simulink model "physical_dynamics_transfer_model"  (R2012b)
settings: Solver=ode1  StartTime=0.0  StopTime=10  FixedStep=0.002  RelTol=1e-3
undefined symbols (not defined in the file or in its folder): HIL, x_init
libraries: quarc_library x4
settings Model: ExtModeTrigDuration=5000  Creator=crbonney  LastModifiedBy=crbonney
settings SolverCC: PositivePriorityOrder=on
settings RTWCC: SystemTargetFile=quarc_win64.tlc  TemplateMakefile=quarc_default_tmf  Description=QUARC Win64 Target  ProcessScript=quarc_win64_make_rtw_hook
settings STFCustomTargetCC: TargetPreCompLibLocation=C:\PROGRA~3\QUARC\lib\2012b\win64\release  CodeReplacementLibrary=ANSI_C  GeneratePreprocessorConditionals=Disable all  CombineOutputUpdateFcns=on  GRTInterface=off  SystemTargetFile=quarc_win64.tlc
settings GRTTargetCC: TargetPreCompLibLocation=C:\PROGRA~3\QUARC\lib\2012b\win64\release  ParMdlRefBuildCompliant=off  CompOptLevelCompliant=off  ConcurrentExecutionCompliant=off  MatFileLogging=off  ExtMode=on  ExtModeMexFile=quarc_comm

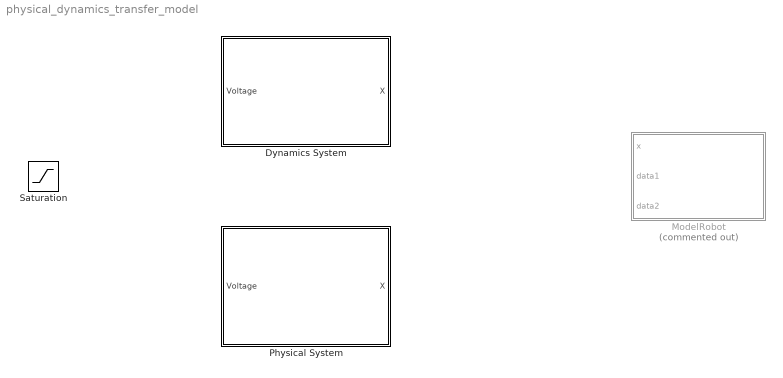
== system physical_dynamics_transfer_model ==
  Dynamics System : Subsystem
  ModelRobot : MATLAB Function  Commented=on  TreatAsAtomicUnit=on
  Physical System : Subsystem
  Saturation : Saturate  UpperLimit=10  LowerLimit=-10
  wires:
  ? -> Saturation/1  "Input V"

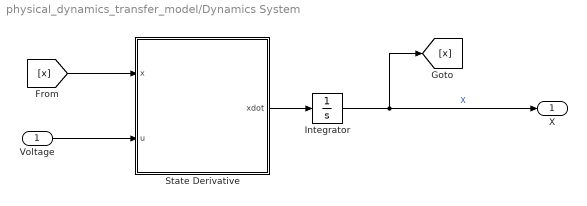
== system physical_dynamics_transfer_model/Dynamics System ==
  Voltage : Inport
  Integrator : Integrator  InitialCondition=x_init
  State Derivative : MATLAB Function  TreatAsAtomicUnit=on
  X : Outport
  wires:
  State Derivative/1(xdot) -> Integrator/1
  Voltage/1 -> State Derivative/2(u)
  [x] -> State Derivative/1(x)
  Integrator/1 -> X/1, [x]  "X"

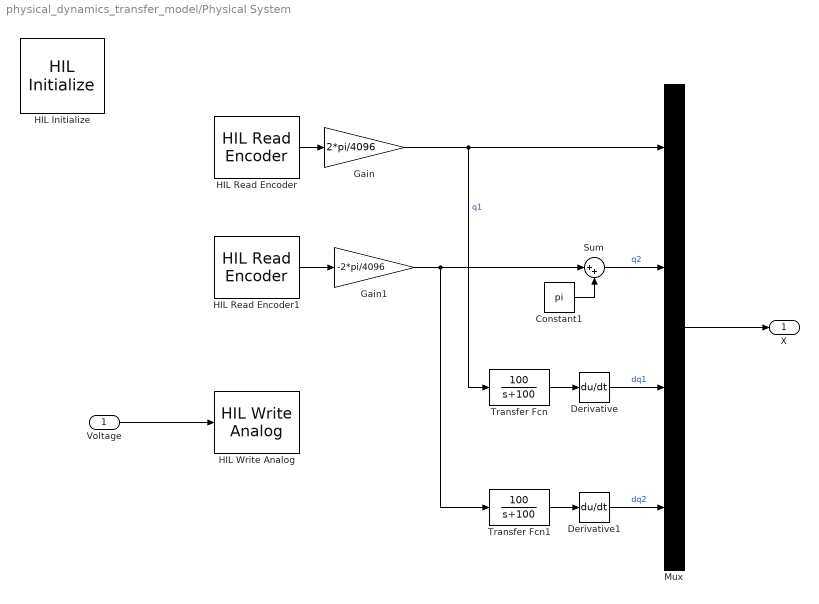
== system physical_dynamics_transfer_model/Physical System ==
  Voltage : Inport
  Constant1 : Constant  Value=pi
  Derivative : Derivative
  Derivative1 : Derivative
  Gain : Gain  Gain=2*pi/4096
  Gain1 : Gain  Gain=-2*pi/4096
  HIL Initialize : quarc_library/Data Acquisition/Generic/Configuration/HIL Initialize  Priority=-99  object_name=HIL-1  board_type=q2_usb  board_number=0  board_options=d0=digital;d1=digital;led=auto;update_rate=normal;decimation=1  exclusive=off  active=off  hardware_clocks=[0]  clock_modes=[]  initial_clock_frequencies=[]  set_clock_params_at_start=off  set_clock_params_at_switch_in=off  set_clock_frequencies_at_start=off  set_clock_frequencies_at_switch_in=off  analog_input_channels=[0:1]  analog_input_maximums=10  analog_input_minimums=-10  set_analog_input_params_at_start=on  set_analog_input_params_at_switch_in=off  analog_output_channels=[0:1]  analog_output_maximums=10  analog_output_minimums=-10  initial_analog_outputs=[0]  final_analog_outputs=[0]  watchdog_analog_outputs=0  set_analog_output_params_at_start=on  set_analog_output_params_at_switch_in=off  set_analog_outputs_at_start=on  set_analog_outputs_at_switch_in=off  set_analog_outputs_at_terminate=on  set_analog_outputs_at_switch_out=off  set_analog_outputs_on_watchdog=off  digital_input_channels=[]  digital_output_channels=[]  digital_output_configuration=[]  initial_digital_outputs=[1]  final_digital_outputs=[1]  watchdog_digital_outputs=[1]  set_digital_output_params_at_start=off  set_digital_output_params_at_switch_in=off  set_digital_outputs_at_start=on  set_digital_outputs_at_switch_in=off  set_digital_outputs_at_terminate=on  set_digital_outputs_at_switch_out=off  set_digital_outputs_on_watchdog=off  encoder_channels=[0:1]  quadrature=[4]  encoder_filter_frequency=[]  initial_encoder_counts=[0]  set_encoder_params_at_start=on  set_encoder_params_at_switch_in=off  set_encoder_counts_at_start=on  set_encoder_counts_at_switch_in=off  pwm_channels=[]  pwm_modes=[0]  pwm_frequency=1/0.020  pwm_configuration=[]  pwm_alignment=[]  pwm_polarity=[]  pwm_leading_deadband=[]  pwm_trailing_deadband=[]  initial_pwm_outputs=[0]  final_pwm_outputs=[0]  watchdog_pwm_outputs=[0]  set_pwm_params_at_start=on  set_pwm_params_at_switch_in=off  set_pwm_outputs_at_start=on  set_pwm_outputs_at_switch_in=off  set_pwm_outputs_at_terminate=on  set_pwm_outputs_at_switch_out=off  set_pwm_outputs_on_watchdog=off  other_output_channels=[]  initial_other_outputs=[]  final_other_outputs=[]  watchdog_other_outputs=[]  set_other_outputs_at_start=off  set_other_outputs_at_switch_in=off  set_other_outputs_at_terminate=off  set_other_outputs_at_switch_out=off  set_other_outputs_on_watchdog=off
  HIL Read Encoder : quarc_library/Data Acquisition/Generic/Immediate I//O/HIL Read Encoder  object_name=HIL-1  channels=0  sample_time=qc_get_step_size  active=on  vector_output=off  data_type_mode=Inherit via back propagation  data_type=double
  HIL Read Encoder1 : quarc_library/Data Acquisition/Generic/Immediate I//O/HIL Read Encoder  object_name=HIL-1  channels=1  sample_time=qc_get_step_size  active=on  vector_output=off  data_type_mode=Inherit via back propagation  data_type=double
  HIL Write Analog : quarc_library/Data Acquisition/Generic/Immediate I//O/HIL Write Analog  object_name=HIL-1  channels=0  sample_time=-1  active=off  vector_input=off
  Mux : Mux
  Sum : Sum  Inputs=|++
  Transfer Fcn : TransferFcn  Numerator=[100]  Denominator=[1 100]
  Transfer Fcn1 : TransferFcn  Numerator=[100]  Denominator=[1 100]
  X : Outport
  wires:
  Voltage/1 -> HIL Write Analog/1
  Derivative1/1 -> Mux/4  "dq2"
  Transfer Fcn1/1 -> Derivative1/1
  Transfer Fcn/1 -> Derivative/1
  Derivative/1 -> Mux/3  "dq1"
  HIL Read Encoder/1 -> Gain/1
  HIL Read Encoder1/1 -> Gain1/1
  Constant1/1 -> Sum/2
  Gain1/1 -> Transfer Fcn1/1, Sum/1
  Gain/1 -> Transfer Fcn/1, Mux/1  "q1"
  Sum/1 -> Mux/2  "q2"
  Mux/1 -> X/1

== matlab function physical_dynamics_transfer_model/ModelRobot ==
  data: x input; data1 input; data2 input
function ModelRobot (x,data1,data2)

theta1 = x(1);
theta2 = x(2);

    frame0_links = ...
        [0  0;...  %X
         0  0;...  %Y
         0 -15];   %Z

    frame1_links = ...
        [0  0  0  0 0;... %X
         0  0  6  6 8;... %Y
         0 -1 -1  0 0];   %Z

    frame2_links = ...
        [0   0;... %X
         0  12;... %Y
         0   0];   %Z

    rho = sqrt(8^2+12^2);
    phi_max = atan(12/8);

    f1 = TransformPoints(TRANS0_1(theta1),frame1_links);
    f2 = TransformPoints(TRANS0_1(theta1),TransformPoints(TRANS1_2(theta2),frame2_links));
    d1 = TransformPoints(TRANS0_1(data1),frame1_links);
    d2 = TransformPoints(TRANS0_1(data1),TransformPoints(TRANS1_2(data2),frame2_links));    

    plot3(frame0_links(1,:),frame0_links(2,:), frame0_links(3,:),'bs-','LineWidth',3);
    axis([-15 15 -15 15 -15 15]);
    grid on
    hold on
    xlabel('x');
    ylabel('y');
    zlabel('z');
    plot3(f1(1,:),f1(2,:), f1(3,:),'rs-','LineWidth',3);
    plot3(f2(1,:),f2(2,:), f2(3,:),'go-', 'MarkerFaceColor', 'c', 'MarkerSize',5,'LineWidth',3);
    plot3(f2(1,end),f2(2,end), f2(3,end),'go-', 'MarkerFaceColor', 'c', 'MarkerSize',5,'LineWidth',3);

    plot3(d1(1,:),d1(2,:), d1(3,:),'ks-','LineWidth',3);
    plot3(d2(1,:),d2(2,:), d2(3,:),'ko-', 'MarkerFaceColor', 'k', 'MarkerSize',5,'LineWidth',3);
    plot3(d2(1,end),d2(2,end), d2(3,end),'ko-', 'MarkerFaceColor', 'k', 'MarkerSize',5,'LineWidth',3);

    axis([-15 15 -15 15 -15 15]);
    WorkEnvelope2(rho, phi_max);
    hold off
end

== matlab function physical_dynamics_transfer_model/Dynamics System/State Derivative ==
  data: x input; u input; xdot output
function xdot = fcn(x, u)

J1 = 0.0012;
m2 = 0.127;
L12 = 0.2;
L2 = 0.3;
Lc2 = L2/2;
beta1 = 0.015;
beta2 = 0.002;
Ra = 2.6;
kt = 0.00768;
kr = 70;
g = 9.81;

theta1 = (J1+m2*L12^2)*Ra/(kr*kt);
theta2 = 1/3*m2*L2^2*Ra/(kr*kt);
theta3 = 1/2*m2*L12*L2*Ra/(kr*kt);
theta4 = m2*Lc2*Ra/(kr*kt);
theta5 = beta1*Ra/(kr*kt)+kr*kt;
theta6 = beta2*Ra/(kr*kt);

q1 = x(1);
q2 = x(2);
q1dot = x(3);
q2dot = x(4);
v = [u; 0];

m =    [...
        (theta1+theta2*sin(q2)^2) (theta3*cos(q2));...
            (theta3*cos(q2)) (theta2);...
];


c =    [...
             (2*theta2*cos(q2)*q2dot) (-theta3*sin(q2)*q2dot);...
         (-theta2*sin(q2)*cos(q2)*q1dot) (0);...
];


f =    [...
         theta5*q1dot;...
         theta6*q2dot;...
];

g =    [...
                  0;...
        -theta4*g*sin(q2);...
];


acceleration = -m\(c*[q1dot;q2dot]+f+g-v);

xdot = [q1dot;q2dot;acceleration];
